simulink model "DC_Motor_PID"  (R2013a)
settings: Solver=ode45  StartTime=0.0  StopTime=3  RelTol=1e-3
values from neighbouring files (symbols this model uses):
  b = 3.5077E-6    (= 3.5077e-06)    [DC_Motor.m]
  J = 3.2284E-6    (= 3.2284e-06)    [DC_Motor.m]
  Kb = 0.0274    [DC_Motor.m]
  Kt = 0.0274    [DC_Motor.m]
  L = 2.75E-6    (= 2.75e-06)    [DC_Motor.m]
  R = 4    [DC_Motor.m]
libraries: simulink x1
settings Model: Creator=DZR3QN  LastModifiedBy=Abhishek
settings DataIOCC: SignalLoggingSaveFormat=ModelDataLogs
settings DebuggingCC: UnderspecifiedInitializationDetection=Simplified  MultiTaskDSMMsg=warning  MultiTaskCondExecSysMsg=none  StateNameClashWarn=none  StrictBusMsg=ErrorOnBusTreatedAsVector
settings RTWCC: IncludeERTFirstTime=on
settings GRTTargetCC: CodeReplacementLibrary=None  CPPClassGenCompliant=on

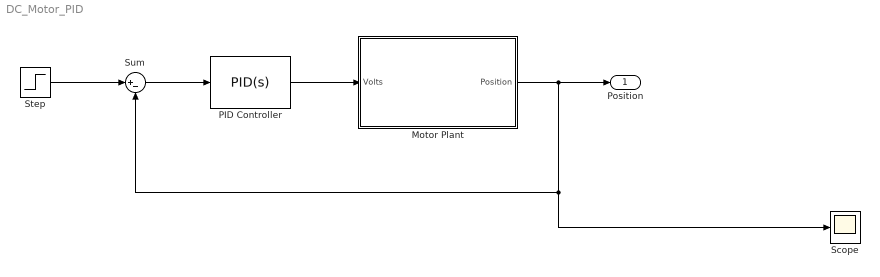
== system DC_Motor_PID ==
  Motor Plant : Subsystem
  PID Controller : simulink/Continuous/PID Controller  Controller=PID  TimeDomain=Continuous-time  SampleTime=1  IntegratorMethod=Forward Euler  FilterMethod=Forward Euler  Form=Parallel  P=1  I=1  D=0  N=100  InitialConditionSource=internal  InitialConditionForIntegrator=0  InitialConditionForFilter=0  ExternalReset=none  LimitOutput=off  UpperSaturationLimit=inf  LowerSaturationLimit=-inf  LinearizeAsGain=on  AntiWindupMode=none  Kb=1  TrackingMode=off  Kt=1  PParamMin=[]  PParamMax=[]  IParamMin=[]  IParamMax=[]  DParamMin=[]  DParamMax=[]  NParamMin=[]  NParamMax=[]  KbParamMin=[]  KbParamMax=[]  KtParamMin=[]  KtParamMax=[]  POutMin=[]  POutMax=[]  IOutMin=[]  IOutMax=[]  DOutMin=[]  DOutMax=[]  NOutMin=[]  NOutMax=[]  KbOutMin=[]  KbOutMax=[]  KtOutMin=[]  KtOutMax=[]  IntegratorOutMin=[]  IntegratorOutMax=[]  FilterOutMin=[]  FilterOutMax=[]  SumOutMin=[]  SumOutMax=[]  SumI1OutMin=[]  SumI1OutMax=[]  SumI2OutMin=[]  SumI2OutMax=[]  SumI3OutMin=[]  SumI3OutMax=[]  SumDOutMin=[]  SumDOutMax=[]  SaturationOutMin=[]  SaturationOutMax=[]  IntegratorContinuousStateAttributes=''  IntegratorStateMustResolveToSignalObject=off  IntegratorRTWStateStorageClass=Auto  FilterContinuousStateAttributes=''  FilterStateMustResolveToSignalObject=off  FilterRTWStateStorageClass=Auto
  Scope : Scope
      settings: MaxDataPoints=50000000
  Step : Step  SampleTime=0
  Sum : Sum  Inputs=|+-
  Position : Outport
  wires:
  Sum/1 -> PID Controller/1
  PID Controller/1 -> Motor Plant/1(Volts)
  Step/1 -> Sum/1
  Motor Plant/1(Position) -> Position/1, Scope/1, Sum/2

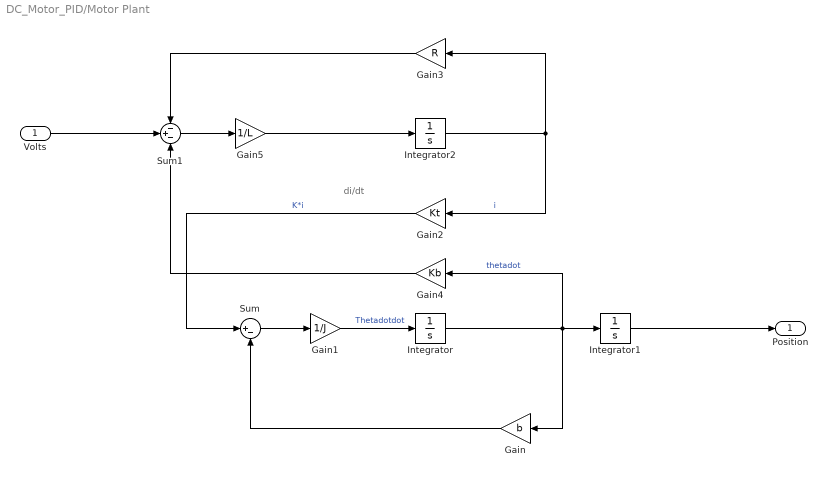
== system DC_Motor_PID/Motor Plant ==
  note: di/dt
  Volts : Inport
  Gain : Gain  Gain=b
  Gain1 : Gain  Gain=1/J
  Gain2 : Gain  Gain=Kt
  Gain3 : Gain  Gain=R
  Gain4 : Gain  Gain=Kb
  Gain5 : Gain  Gain=1/L
  Integrator : Integrator
  Integrator1 : Integrator
  Integrator2 : Integrator
  Sum : Sum  Inputs=|+-
  Sum1 : Sum  Inputs=-+-
  Position : Outport
  wires:
  Gain/1 -> Sum/2
  Gain5/1 -> Integrator2/1
  Integrator2/1 -> Gain2/1, Gain3/1  "i"
  Sum/1 -> Gain1/1
  Gain3/1 -> Sum1/1
  Gain2/1 -> Sum/1  "K*i"
  Volts/1 -> Sum1/2
  Gain4/1 -> Sum1/3
  Sum1/1 -> Gain5/1
  Gain1/1 -> Integrator/1  "Thetadotdot"
  Integrator1/1 -> Position/1
  Integrator/1 -> Gain4/1, Gain/1, Integrator1/1  "thetadot"
